simulink model "DY05S600_robot_controller_main_opensource"  (R2020a)
settings: Solver=FixedStepAuto  StartTime=0.0  StopTime=inf  FixedStep=SAMPLE_TIME  RelTol=1e-3
(part 1 of 2)
settings Model: ExplicitPartitioning=on  Creator=86166  LastModifiedBy=win
settings OptimizationCC: BlockReduction=off  EnhancedBackFolding=on  PassReuseOutputArgsThreshold=0  OptimizeBlockOrder=speed  DifferentSizesBufferReuse=on  OptimizationCustomize=off
settings DebuggingCC: ParameterTunabilityLossMsg=error
settings HardwareCC: ProdBitPerLong=64  ProdHWDeviceType=Intel->x86-64 (Linux 64)  TargetBitPerPointer=64  TargetBitPerSizeT=64  TargetBitPerPtrDiffT=64  TargetLongLongMode=on  TargetIntDivRoundTo=Zero  TargetEndianess=LittleEndian  TargetWordSize=64  TargetHWDeviceType=Custom Processor->MATLAB Host Computer
settings RTWCC: Description=Generic Real-Time Target  SystemTargetFile=links_rtlnx_grt.tlc  GenCodeOnly=on  TemplateMakefile=links_rtlnx_grt.tmf  GenerateReport=on  RTWVerbose=off  CustomLibrary=libethercat.a  LaunchReport=on
settings CodeAppCC: ForceParamTrailComments=on  OperatorAnnotations=on
settings STFCustomTargetCC: ModelReferenceCompliant=off  CombineOutputUpdateFcns=on  SystemTargetFile=links_rtlnx_grt.tlc
settings GRTTargetCC: TargetLangStandard=C89/C90 (ANSI)  ModelReferenceCompliant=off  ParMdlRefBuildCompliant=off  CompOptLevelCompliant=off  ConcurrentExecutionCompliant=off  MatFileLogging=off  CPPClassGenCompliant=off  UseToolchainInfoCompliant=off  RTWCAPISignals=on  RTWCAPIParams=on  RTWCAPIRootIO=on

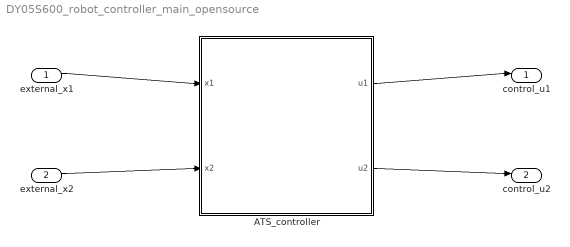
== system DY05S600_robot_controller_main_opensource ==
  external_x1 : Inport
  external_x2 : Inport  Port=2
  ATS_controller : Subsystem
  control_u1 : Outport
  control_u2 : Outport  Port=2
  wires:
  external_x1/1 -> ATS_controller/1(x1)
  external_x2/1 -> ATS_controller/2(x2)
  ATS_controller/1(u1) -> control_u1/1
  ATS_controller/2(u2) -> control_u2/1

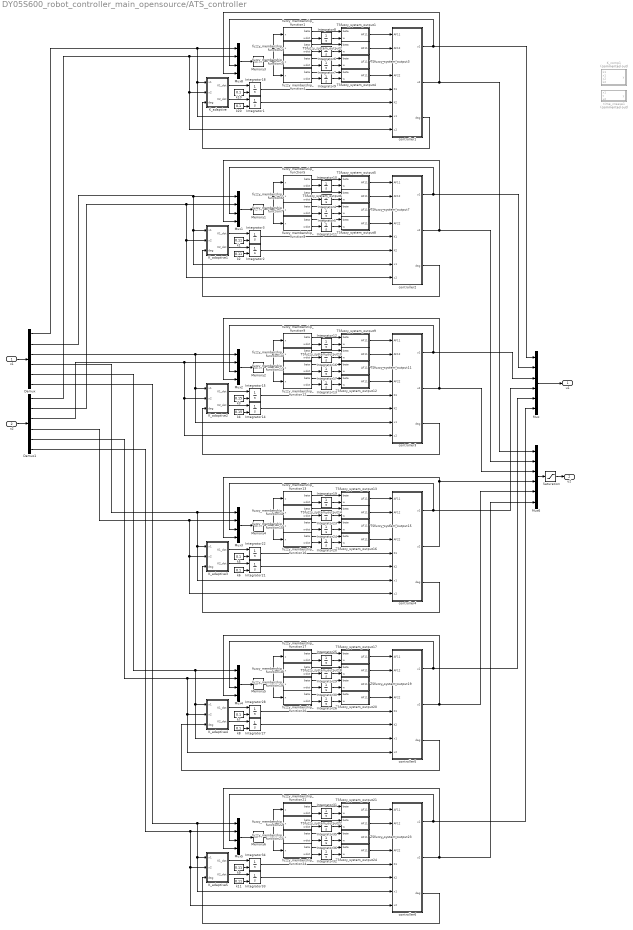
== system DY05S600_robot_controller_main_opensource/ATS_controller ==
  x1 : Inport
  x2 : Inport  Port=2
  Demux : Demux  Outputs=6
  Demux1 : Demux  Outputs=6
  Integrator{1..3,14..15,18,21..22,27..28,33..34} (12 alike) : Integrator  InitialConditionSource=external
  Integrator{4..13,16..17,19..20,23..26,29..32,35..36} (24 alike) : Integrator
  K_adaptive : MATLAB Function  TreatAsAtomicUnit=on
  K_adaptive1 : MATLAB Function  TreatAsAtomicUnit=on
  K_adaptive2 : MATLAB Function  TreatAsAtomicUnit=on
  K_adaptive3 : MATLAB Function  TreatAsAtomicUnit=on
  K_adaptive4 : MATLAB Function  TreatAsAtomicUnit=on
  K_adaptive5 : MATLAB Function  TreatAsAtomicUnit=on
  K_comp1 : MATLAB Function  Commented=on  TreatAsAtomicUnit=on
  Memory{1..6} (6 alike) : Memory
  Mux : Mux  Inputs=6
  Mux{1..5,8} (6 alike) : Mux
  Mux6 : Mux  Inputs=6
  Saturation : Saturate  UpperLimit=80  LowerLimit=-80
  TSfuzzy_system_output1 : MATLAB Function  TreatAsAtomicUnit=on
  TSfuzzy_system_output10 : MATLAB Function  TreatAsAtomicUnit=on
  TSfuzzy_system_output11 : MATLAB Function  TreatAsAtomicUnit=on
  TSfuzzy_system_output12 : MATLAB Function  TreatAsAtomicUnit=on
  TSfuzzy_system_output13 : MATLAB Function  TreatAsAtomicUnit=on
  TSfuzzy_system_output14 : MATLAB Function  TreatAsAtomicUnit=on
  TSfuzzy_system_output15 : MATLAB Function  TreatAsAtomicUnit=on
  TSfuzzy_system_output16 : MATLAB Function  TreatAsAtomicUnit=on
  TSfuzzy_system_output17 : MATLAB Function  TreatAsAtomicUnit=on
  TSfuzzy_system_output18 : MATLAB Function  TreatAsAtomicUnit=on
  TSfuzzy_system_output19 : MATLAB Function  TreatAsAtomicUnit=on
  TSfuzzy_system_output2 : MATLAB Function  TreatAsAtomicUnit=on
  TSfuzzy_system_output20 : MATLAB Function  TreatAsAtomicUnit=on
  TSfuzzy_system_output21 : MATLAB Function  TreatAsAtomicUnit=on
  TSfuzzy_system_output22 : MATLAB Function  TreatAsAtomicUnit=on
  TSfuzzy_system_output23 : MATLAB Function  TreatAsAtomicUnit=on
  TSfuzzy_system_output24 : MATLAB Function  TreatAsAtomicUnit=on
  TSfuzzy_system_output3 : MATLAB Function  TreatAsAtomicUnit=on
  TSfuzzy_system_output4 : MATLAB Function  TreatAsAtomicUnit=on
  TSfuzzy_system_output5 : MATLAB Function  TreatAsAtomicUnit=on
  TSfuzzy_system_output6 : MATLAB Function  TreatAsAtomicUnit=on
  TSfuzzy_system_output7 : MATLAB Function  TreatAsAtomicUnit=on
  TSfuzzy_system_output8 : MATLAB Function  TreatAsAtomicUnit=on
  TSfuzzy_system_output9 : MATLAB Function  TreatAsAtomicUnit=on
  controller1 : MATLAB Function  TreatAsAtomicUnit=on
  controller2 : MATLAB Function  TreatAsAtomicUnit=on
  controller3 : MATLAB Function  TreatAsAtomicUnit=on
  controller4 : MATLAB Function  TreatAsAtomicUnit=on
  controller5 : MATLAB Function  TreatAsAtomicUnit=on
  controller6 : MATLAB Function  TreatAsAtomicUnit=on
  fuzzy_membership_function1 : MATLAB Function  TreatAsAtomicUnit=on
  fuzzy_membership_function10 : MATLAB Function  TreatAsAtomicUnit=on
  fuzzy_membership_function11 : MATLAB Function  TreatAsAtomicUnit=on
  fuzzy_membership_function12 : MATLAB Function  TreatAsAtomicUnit=on
  fuzzy_membership_function13 : MATLAB Function  TreatAsAtomicUnit=on
  fuzzy_membership_function14 : MATLAB Function  TreatAsAtomicUnit=on
  fuzzy_membership_function15 : MATLAB Function  TreatAsAtomicUnit=on
  fuzzy_membership_function16 : MATLAB Function  TreatAsAtomicUnit=on
  fuzzy_membership_function17 : MATLAB Function  TreatAsAtomicUnit=on
  fuzzy_membership_function18 : MATLAB Function  TreatAsAtomicUnit=on
  fuzzy_membership_function19 : MATLAB Function  TreatAsAtomicUnit=on
  fuzzy_membership_function2 : MATLAB Function  TreatAsAtomicUnit=on
  fuzzy_membership_function20 : MATLAB Function  TreatAsAtomicUnit=on
  fuzzy_membership_function21 : MATLAB Function  TreatAsAtomicUnit=on
  fuzzy_membership_function22 : MATLAB Function  TreatAsAtomicUnit=on
  fuzzy_membership_function23 : MATLAB Function  TreatAsAtomicUnit=on
  fuzzy_membership_function24 : MATLAB Function  TreatAsAtomicUnit=on
  fuzzy_membership_function3 : MATLAB Function  TreatAsAtomicUnit=on
  fuzzy_membership_function4 : MATLAB Function  TreatAsAtomicUnit=on
  fuzzy_membership_function5 : MATLAB Function  TreatAsAtomicUnit=on
  fuzzy_membership_function6 : MATLAB Function  TreatAsAtomicUnit=on
  fuzzy_membership_function7 : MATLAB Function  TreatAsAtomicUnit=on
  fuzzy_membership_function8 : MATLAB Function  TreatAsAtomicUnit=on
  fuzzy_membership_function9 : MATLAB Function  TreatAsAtomicUnit=on
  k{1..2,9,11} (4 alike) : Constant  Value=0.11  VectorParams1D=off  SampleTime=-1
  k{5..8,10,20} (6 alike) : Constant  Value=0.1  VectorParams1D=off  SampleTime=-1
  k3 : Constant  Value=0.15  VectorParams1D=off  SampleTime=-1
  k4 : Constant  Value=0.15  VectorParams1D=off  SampleTime=-1
  time_crease1 : MATLAB Function  Commented=on  TreatAsAtomicUnit=on
  u1 : Outport
  u2 : Outport  Port=2
  wires:
  TSfuzzy_system_output1/1(AF11) -> controller1/1(AF11)
  k20/1 -> Integrator1/2
  Memory3/1 -> fuzzy_membership_function4/1(x), fuzzy_membership_function3/1(x), fuzzy_membership_function2/1(x), fuzzy_membership_function1/1(x)
  K_adaptive/2(K2_dot) -> Integrator1/1
  Integrator6/1 -> TSfuzzy_system_output2/2(w)
  Mux8/1 -> Memory3/1
  controller1/1(u1) -> Mux8/3, Mux/1
  TSfuzzy_system_output4/1(AF11) -> controller1/4(AF22)
  Integrator8/1 -> TSfuzzy_system_output1/2(w)
  fuzzy_membership_function1/1(beta) -> TSfuzzy_system_output1/1(beta)
  fuzzy_membership_function2/1(beta) -> TSfuzzy_system_output2/1(beta)
  Integrator9/1 -> TSfuzzy_system_output4/2(w)
  fuzzy_membership_function4/1(beta) -> TSfuzzy_system_output4/1(beta)
  fuzzy_membership_function1/2(wdot) -> Integrator8/1
  fuzzy_membership_function2/2(wdot) -> Integrator6/1
  K_adaptive/1(K1_dot) -> Integrator18/1
  Integrator7/1 -> TSfuzzy_system_output3/2(w)
  TSfuzzy_system_output2/1(AF11) -> controller1/2(AF12)
  fuzzy_membership_function3/2(wdot) -> Integrator7/1
  fuzzy_membership_function4/2(wdot) -> Integrator9/1
  TSfuzzy_system_output3/1(AF11) -> controller1/3(AF21)
  k10/1 -> Integrator18/2
  fuzzy_membership_function3/1(beta) -> TSfuzzy_system_output3/1(beta)
  x1/1 -> Demux/1
  x2/1 -> Demux1/1
  Demux1/1 -> controller1/8(x2), K_adaptive/2(x2), Mux8/2
  controller1/3(dag) -> K_adaptive/3(dag)
  fuzzy_membership_function7/1(beta) -> TSfuzzy_system_output7/1(beta)
  k1/1 -> Integrator3/2
  fuzzy_membership_function8/2(wdot) -> Integrator11/1
  TSfuzzy_system_output7/1(AF11) -> controller2/3(AF21)
  fuzzy_membership_function7/2(wdot) -> Integrator5/1
  fuzzy_membership_function5/2(wdot) -> Integrator10/1
  TSfuzzy_system_output6/1(AF11) -> controller2/2(AF12)
  K_adaptive1/1(K1_dot) -> Integrator3/1
  Integrator5/1 -> TSfuzzy_system_output7/2(w)
  Integrator11/1 -> TSfuzzy_system_output8/2(w)
  fuzzy_membership_function8/1(beta) -> TSfuzzy_system_output8/1(beta)
  fuzzy_membership_function6/1(beta) -> TSfuzzy_system_output6/1(beta)
  controller2/1(u1) -> Mux1/3, Mux/2
  Mux1/1 -> Memory1/1
  fuzzy_membership_function5/1(beta) -> TSfuzzy_system_output5/1(beta)
  controller2/2(u2) -> Mux1/4, Mux6/2
  K_adaptive1/2(K2_dot) -> Integrator2/1
  Integrator10/1 -> TSfuzzy_system_output5/2(w)
  k2/1 -> Integrator2/2
  Integrator4/1 -> TSfuzzy_system_output6/2(w)
  controller2/3(dag) -> K_adaptive1/3(dag)
  Memory1/1 -> fuzzy_membership_function8/1(x), fuzzy_membership_function7/1(x), fuzzy_membership_function6/1(x), fuzzy_membership_function5/1(x)
  fuzzy_membership_function6/2(wdot) -> Integrator4/1
  TSfuzzy_system_output5/1(AF11) -> controller2/1(AF11)
  TSfuzzy_system_output8/1(AF11) -> controller2/4(AF22)
  fuzzy_membership_function9/1(beta) -> TSfuzzy_system_output9/1(beta)
  TSfuzzy_system_output12/1(AF11) -> controller3/4(AF22)
  TSfuzzy_system_output9/1(AF11) -> controller3/1(AF11)
  Memory2/1 -> fuzzy_membership_function12/1(x), fuzzy_membership_function11/1(x), fuzzy_membership_function10/1(x), fuzzy_membership_function9/1(x)
  fuzzy_membership_function10/2(wdot) -> Integrator16/1
  Integrator12/1 -> TSfuzzy_system_output9/2(w)
  Integrator16/1 -> TSfuzzy_system_output10/2(w)
  controller3/2(u2) -> Mux2/4, Mux6/3
  fuzzy_membership_function10/1(beta) -> TSfuzzy_system_output10/1(beta)
  Mux2/1 -> Memory2/1
  fuzzy_membership_function11/2(wdot) -> Integrator17/1
  fuzzy_membership_function9/2(wdot) -> Integrator12/1
  TSfuzzy_system_output11/1(AF11) -> controller3/3(AF21)
  TSfuzzy_system_output10/1(AF11) -> controller3/2(AF12)
  fuzzy_membership_function12/2(wdot) -> Integrator13/1
  fuzzy_membership_function12/1(beta) -> TSfuzzy_system_output12/1(beta)
  Integrator17/1 -> TSfuzzy_system_output11/2(w)
  controller3/1(u1) -> Mux2/3, Mux/3
  K_adaptive2/1(K1_dot) -> Integrator15/1
  fuzzy_membership_function11/1(beta) -> TSfuzzy_system_output11/1(beta)
  Integrator13/1 -> TSfuzzy_system_output12/2(w)
  fuzzy_membership_function13/1(beta) -> TSfuzzy_system_output13/1(beta)
  TSfuzzy_system_output16/1(AF11) -> controller4/4(AF22)
  TSfuzzy_system_output13/1(AF11) -> controller4/1(AF11)
  Memory4/1 -> fuzzy_membership_function16/1(x), fuzzy_membership_function15/1(x), fuzzy_membership_function14/1(x), fuzzy_membership_function13/1(x)
  fuzzy_membership_function14/2(wdot) -> Integrator23/1
  Integrator19/1 -> TSfuzzy_system_output13/2(w)
  controller4/3(dag) -> K_adaptive3/3(dag)
  Integrator23/1 -> TSfuzzy_system_output14/2(w)
  controller4/2(u2) -> Mux6/4, Mux3/4
  fuzzy_membership_function14/1(beta) -> TSfuzzy_system_output14/1(beta)
  Mux3/1 -> Memory4/1
  fuzzy_membership_function15/2(wdot) -> Integrator24/1
  fuzzy_membership_function13/2(wdot) -> Integrator19/1
  TSfuzzy_system_output15/1(AF11) -> controller4/3(AF21)
  TSfuzzy_system_output14/1(AF11) -> controller4/2(AF12)
  fuzzy_membership_function16/2(wdot) -> Integrator20/1
  fuzzy_membership_function16/1(beta) -> TSfuzzy_system_output16/1(beta)
  Integrator24/1 -> TSfuzzy_system_output15/2(w)
  controller4/1(u1) -> Mux/4, Mux3/3
  K_adaptive3/1(K1_dot) -> Integrator22/1
  fuzzy_membership_function15/1(beta) -> TSfuzzy_system_output15/1(beta)
  Integrator20/1 -> TSfuzzy_system_output16/2(w)
  fuzzy_membership_function17/1(beta) -> TSfuzzy_system_output17/1(beta)
  TSfuzzy_system_output20/1(AF11) -> controller5/4(AF22)
  TSfuzzy_system_output17/1(AF11) -> controller5/1(AF11)
  Memory5/1 -> fuzzy_membership_function20/1(x), fuzzy_membership_function19/1(x), fuzzy_membership_function18/1(x), fuzzy_membership_function17/1(x)
  fuzzy_membership_function18/2(wdot) -> Integrator29/1
  Integrator25/1 -> TSfuzzy_system_output17/2(w)
  controller5/3(dag) -> K_adaptive4/3(dag)
  Integrator29/1 -> TSfuzzy_system_output18/2(w)
  controller5/2(u2) -> Mux6/5, Mux4/4
  fuzzy_membership_function18/1(beta) -> TSfuzzy_system_output18/1(beta)
  Mux4/1 -> Memory5/1
  fuzzy_membership_function19/2(wdot) -> Integrator30/1
  fuzzy_membership_function17/2(wdot) -> Integrator25/1
  TSfuzzy_system_output19/1(AF11) -> controller5/3(AF21)
  TSfuzzy_system_output18/1(AF11) -> controller5/2(AF12)
  fuzzy_membership_function20/2(wdot) -> Integrator26/1
  fuzzy_membership_function20/1(beta) -> TSfuzzy_system_output20/1(beta)
  Integrator30/1 -> TSfuzzy_system_output19/2(w)
  controller5/1(u1) -> Mux/5, Mux4/3
  K_adaptive4/1(K1_dot) -> Integrator28/1
  fuzzy_membership_function19/1(beta) -> TSfuzzy_system_output19/1(beta)
  Integrator26/1 -> TSfuzzy_system_output20/2(w)
  fuzzy_membership_function21/1(beta) -> TSfuzzy_system_output21/1(beta)
  TSfuzzy_system_output24/1(AF11) -> controller6/4(AF22)
  TSfuzzy_system_output21/1(AF11) -> controller6/1(AF11)
  Memory6/1 -> fuzzy_membership_function24/1(x), fuzzy_membership_function23/1(x), fuzzy_membership_function22/1(x), fuzzy_membership_function21/1(x)
  fuzzy_membership_function22/2(wdot) -> Integrator35/1
  Integrator31/1 -> TSfuzzy_system_output21/2(w)
  controller6/3(dag) -> K_adaptive5/3(dag)
  Integrator35/1 -> TSfuzzy_system_output22/2(w)
  fuzzy_membership_function22/1(beta) -> TSfuzzy_system_output22/1(beta)
  Mux5/1 -> Memory6/1
  fuzzy_membership_function23/2(wdot) -> Integrator36/1
  fuzzy_membership_function21/2(wdot) -> Integrator31/1
  TSfuzzy_system_output23/1(AF11) -> controller6/3(AF21)
  TSfuzzy_system_output22/1(AF11) -> controller6/2(AF12)
  fuzzy_membership_function24/2(wdot) -> Integrator32/1
  fuzzy_membership_function24/1(beta) -> TSfuzzy_system_output24/1(beta)
  Integrator36/1 -> TSfuzzy_system_output23/2(w)
  controller6/1(u1) -> Mux5/3, Mux/6
  K_adaptive5/1(K1_dot) -> Integrator34/1
  fuzzy_membership_function23/1(beta) -> TSfuzzy_system_output23/1(beta)
  Integrator32/1 -> TSfuzzy_system_output24/2(w)
  Demux/2 -> controller2/7(x1), K_adaptive1/1(x1), Mux1/1
  Demux1/2 -> controller2/8(x2), K_adaptive1/2(x2), Mux1/2
  Demux1/3 -> K_adaptive2/2(x2), controller3/8(x2), Mux2/2
  Demux/4 -> K_adaptive3/1(x1), controller4/7(x1), Mux3/1
  Demux1/4 -> K_adaptive3/2(x2), controller4/8(x2), Mux3/2
  Demux/5 -> K_adaptive4/1(x1), controller5/7(x1), Mux4/1
  Demux1/5 -> K_adaptive4/2(x2), controller5/8(x2), Mux4/2
  Demux/6 -> K_adaptive5/1(x1), controller6/7(x1), Mux5/1
  Demux1/6 -> K_adaptive5/2(x2), controller6/8(x2), Mux5/2
  Mux/1 -> u1/1
  Mux6/1 -> Saturation/1
  Saturation/1 -> u2/1
  Integrator3/1 -> controller2/5(K1)
  Integrator2/1 -> controller2/6(K2)
  Integrator15/1 -> controller3/5(K1)
  k4/1 -> Integrator14/2
  Integrator14/1 -> controller3/6(K2)
  K_adaptive2/2(K2_dot) -> Integrator14/1
  k3/1 -> Integrator15/2
  k6/1 -> Integrator21/2
  k5/1 -> Integrator22/2
  Integrator21/1 -> controller4/6(K2)
  K_adaptive3/2(K2_dot) -> Integrator21/1
  Integrator22/1 -> controller4/5(K1)
  Demux/3 -> controller3/7(x1), K_adaptive2/1(x1), Mux2/1
  controller3/3(dag) -> K_adaptive2/3(dag)
  K_adaptive4/2(K2_dot) -> Integrator27/1
  k7/1 -> Integrator28/2
  k8/1 -> Integrator27/2
  Integrator27/1 -> controller5/6(K2)
  Integrator28/1 -> controller5/5(K1)
  K_adaptive5/2(K2_dot) -> Integrator33/1
  k9/1 -> Integrator34/2
  k11/1 -> Integrator33/2
  controller6/2(u2) -> Mux6/6, Mux5/4
  controller1/2(u2) -> Mux6/1, Mux8/4
  Demux/1 -> controller1/7(x1), K_adaptive/1(x1), Mux8/1
  Integrator18/1 -> controller1/5(K1)
  Integrator1/1 -> controller1/6(K2)
  Integrator34/1 -> controller6/5(K1)
  Integrator33/1 -> controller6/6(K2)

== matlab function DY05S600_robot_controller_main_opensource/ATS_controller/fuzzy_membership_function22 ==
  data: x input; beta output; wdot output
function [beta,wdot] = fcn(x)

%xm是规则中心
xm=zeros(5,4);
for j=1:5
    xm(j,1)=-0.26+0.13*(j-1)+0.1;
end
for j=6:10
    xm(j-5,2)=-0.18+0.09*(j-5-1)+0.1;
end
for j=11:15
    xm(j-10,3)=-0.14+0.07*(j-10-1)+0.1;
end
for j=16:20
    xm(j-15,4)=-0.4+0.2*(j-15-1)+0.1;
end



%xm是规则中心从小值到大值排列,x是前件变量,
r=length(xm(:,1)); %length(xm)是规则数量r
n=length(xm(1,:));%length(x)是前件变量维度
%初始化隶属度函数
ux=zeros(r,n);

for k=1:n
    if x(k)<=xm(1,k)   %论域左边界外
        ux(1,k)=1;
    end
    if x(k)>=xm(r,k)   %论域右边界外
        ux(r,k)=1;
    end
    for i=1:r-1  %从左到右只计算下降的隶属度函数
        if x(k)>=xm(i,k)&&x(k)<=xm(i+1,k)
           ux(i,k)=0.5*sin(pi*(x(k)-xm(i,k))/abs(xm(i,k)-xm(i+1,k))+0.5*pi)+0.5; %一种具有一阶可导性的四边形家族隶属度函数
        end
    end
    for i=2:r  %从左到右只计算上升的隶属度函数
        if x(k)>=xm(i-1,k)&&x(k)<=xm(i,k)
           ux(i,k)=0.5*sin(pi*(x(k)-xm(i,k))/abs(xm(i-1,k)-xm(i,k))+0.5*pi)+0.5;
        end
    end
end

kx=1;
jz=1;
[beta,wdot]= fuzzyoutput(ux,x,xm,kx,jz);

% function  [Basic,beta]= sumfuzzy_test(x) 
% ux=x;
% im=1;
% jm=0;
% bias=1;
% Basic=0;
% dem=length(ux(:,1))^length(ux(1,:)); %隶属度函数的重数数量
% beta=zeros(dem,1);
% [Basic,beta] = myfun(im,jm,ux,bias,Basic,beta);
% function [Basic,beta,jm] = myfun(im,jm,ux,bias,Basic,beta) 
% %针对ux隶属度函数矩阵的中心平均解模糊，初值赋为1,0，ux，1，0，执行的是多重求和
%     if  im > length(ux(1,:))    %length(ux(1,:))为前件输入的维度
%         Basic = Basic + bias;
%         jm=jm+1;                %相对于i1...in规则编号，此处是从最后一列填满到第一列（i1,...,in）
%         beta(jm,1)=bias;        %beta(i1,...,in)*xk*z(i6,j)
%     else
%         for km=1:length(ux(:,1))   %length(ux(:,1))为规则数量
%             bias_last = bias;
%             bias = bias* ux(km,im);
%             im = im+1;
%             [Basic,beta,jm] = myfun(im,jm,ux,bias,Basic,beta); %递归，拦在这里一直到function执行结束,每执行一次就会多一个for循环（每次跳出就是再一次的for内循环）
%             im = im-1; 
%             bias  = bias_last;
%         end
%     end
% end


end

== matlab function DY05S600_robot_controller_main_opensource/ATS_controller/fuzzy_membership_function23 ==
  data: x input; beta output; wdot output
function [beta,wdot] = fcn(x)

%xm是规则中心
xm=zeros(5,4);
for j=1:5
    xm(j,1)=-0.26+0.13*(j-1)+0.1;
end
for j=6:10
    xm(j-5,2)=-0.18+0.09*(j-5-1)+0.1;
end
for j=11:15
    xm(j-10,3)=-0.14+0.07*(j-10-1)+0.1;
end
for j=16:20
    xm(j-15,4)=-0.4+0.2*(j-15-1)+0.1;
end


%xm是规则中心从小值到大值排列,x是前件变量,
r=length(xm(:,1)); %length(xm)是规则数量r
n=length(xm(1,:));%length(x)是前件变量维度
%初始化隶属度函数
ux=zeros(r,n);

for k=1:n
    if x(k)<=xm(1,k)   %论域左边界外
        ux(1,k)=1;
    end
    if x(k)>=xm(r,k)   %论域右边界外
        ux(r,k)=1;
    end
    for i=1:r-1  %从左到右只计算下降的隶属度函数
        if x(k)>=xm(i,k)&&x(k)<=xm(i+1,k)
           ux(i,k)=0.5*sin(pi*(x(k)-xm(i,k))/abs(xm(i,k)-xm(i+1,k))+0.5*pi)+0.5; %一种具有一阶可导性的四边形家族隶属度函数
        end
    end
    for i=2:r  %从左到右只计算上升的隶属度函数
        if x(k)>=xm(i-1,k)&&x(k)<=xm(i,k)
           ux(i,k)=0.5*sin(pi*(x(k)-xm(i,k))/abs(xm(i-1,k)-xm(i,k))+0.5*pi)+0.5;
        end
    end
end

kx=1;
jz=1;
[beta,wdot]= fuzzyoutput(ux,x,xm,kx,jz);

% function  [Basic,beta]= sumfuzzy_test(x) 
% ux=x;
% im=1;
% jm=0;
% bias=1;
% Basic=0;
% dem=length(ux(:,1))^length(ux(1,:)); %隶属度函数的重数数量
% beta=zeros(dem,1);
% [Basic,beta] = myfun(im,jm,ux,bias,Basic,beta);
% function [Basic,beta,jm] = myfun(im,jm,ux,bias,Basic,beta) 
% %针对ux隶属度函数矩阵的中心平均解模糊，初值赋为1,0，ux，1，0，执行的是多重求和
%     if  im > length(ux(1,:))    %length(ux(1,:))为前件输入的维度
%         Basic = Basic + bias;
%         jm=jm+1;                %相对于i1...in规则编号，此处是从最后一列填满到第一列（i1,...,in）
%         beta(jm,1)=bias;        %beta(i1,...,in)*xk*z(i6,j)
%     else
%         for km=1:length(ux(:,1))   %length(ux(:,1))为规则数量
%             bias_last = bias;
%             bias = bias* ux(km,im);
%             im = im+1;
%             [Basic,beta,jm] = myfun(im,jm,ux,bias,Basic,beta); %递归，拦在这里一直到function执行结束,每执行一次就会多一个for循环（每次跳出就是再一次的for内循环）
%             im = im-1; 
%             bias  = bias_last;
%         end
%     end
% end


end

== matlab function DY05S600_robot_controller_main_opensource/ATS_controller/fuzzy_membership_function24 ==
  data: x input; beta output; wdot output
function [beta,wdot] = fcn(x)

%xm是规则中心
xm=zeros(5,4);
for j=1:5
    xm(j,1)=-0.26+0.13*(j-1)+0.1;
end
for j=6:10
    xm(j-5,2)=-0.18+0.09*(j-5-1)+0.1;
end
for j=11:15
    xm(j-10,3)=-0.14+0.07*(j-10-1)+0.1;
end
for j=16:20
    xm(j-15,4)=-0.4+0.2*(j-15-1)+0.1;
end



%xm是规则中心从小值到大值排列,x是前件变量,
r=length(xm(:,1)); %length(xm)是规则数量r
n=length(xm(1,:));%length(x)是前件变量维度
%初始化隶属度函数
ux=zeros(r,n);

for k=1:n
    if x(k)<=xm(1,k)   %论域左边界外
        ux(1,k)=1;
    end
    if x(k)>=xm(r,k)   %论域右边界外
        ux(r,k)=1;
    end
    for i=1:r-1  %从左到右只计算下降的隶属度函数
        if x(k)>=xm(i,k)&&x(k)<=xm(i+1,k)
           ux(i,k)=0.5*sin(pi*(x(k)-xm(i,k))/abs(xm(i,k)-xm(i+1,k))+0.5*pi)+0.5; %一种具有一阶可导性的四边形家族隶属度函数
        end
    end
    for i=2:r  %从左到右只计算上升的隶属度函数
        if x(k)>=xm(i-1,k)&&x(k)<=xm(i,k)
           ux(i,k)=0.5*sin(pi*(x(k)-xm(i,k))/abs(xm(i-1,k)-xm(i,k))+0.5*pi)+0.5;
        end
    end
end

kx=1;
jz=1;
[beta,wdot]= fuzzyoutput(ux,x,xm,kx,jz);

% function  [Basic,beta]= sumfuzzy_test(x) 
% ux=x;
% im=1;
% jm=0;
% bias=1;
% Basic=0;
% dem=length(ux(:,1))^length(ux(1,:)); %隶属度函数的重数数量
% beta=zeros(dem,1);
% [Basic,beta] = myfun(im,jm,ux,bias,Basic,beta);
% function [Basic,beta,jm] = myfun(im,jm,ux,bias,Basic,beta) 
% %针对ux隶属度函数矩阵的中心平均解模糊，初值赋为1,0，ux，1，0，执行的是多重求和
%     if  im > length(ux(1,:))    %length(ux(1,:))为前件输入的维度
%         Basic = Basic + bias;
%         jm=jm+1;                %相对于i1...in规则编号，此处是从最后一列填满到第一列（i1,...,in）
%         beta(jm,1)=bias;        %beta(i1,...,in)*xk*z(i6,j)
%     else
%         for km=1:length(ux(:,1))   %length(ux(:,1))为规则数量
%             bias_last = bias;
%             bias = bias* ux(km,im);
%             im = im+1;
%             [Basic,beta,jm] = myfun(im,jm,ux,bias,Basic,beta); %递归，拦在这里一直到function执行结束,每执行一次就会多一个for循环（每次跳出就是再一次的for内循环）
%             im = im-1; 
%             bias  = bias_last;
%         end
%     end
% end


end

== matlab function DY05S600_robot_controller_main_opensource/ATS_controller/K_adaptive3 ==
  data: K1_dot output; x1 input; x2 input; dag input; K2_dot output
function [K1_dot,K2_dot]  = fcn(x1,x2,dag)
w1=0.0001;
w2=0.0001;
K1_dot=w1*x1*4/pi*atan(x1/dag);
K2_dot=w2*x2*4/pi*atan(x2/dag);
end

== matlab function DY05S600_robot_controller_main_opensource/ATS_controller/time_crease1 ==
  data: y output; x1 input; t input; x2 input
function y   = fcn(x1,t,x2)
y1=2/pi*(atan(2*t-1)+pi/4)*x1;
y2=2/pi*(atan(2*t-1)+pi/4)*x2;
y=[y1,y2]';
end

== matlab function DY05S600_robot_controller_main_opensource/ATS_controller/K_adaptive4 ==
  data: K1_dot output; x1 input; x2 input; dag input; K2_dot output
function [K1_dot,K2_dot]  = fcn(x1,x2,dag)
w1=0.0001;
w2=0.0001;
K1_dot=w1*x1*4/pi*atan(x1/dag);
K2_dot=w2*x2*4/pi*atan(x2/dag);
end

== matlab function DY05S600_robot_controller_main_opensource/ATS_controller/K_adaptive5 ==
  data: K1_dot output; x1 input; x2 input; dag input; K2_dot output
function [K1_dot,K2_dot]  = fcn(x1,x2,dag)

w1=0.0001;
w2=0.0001;

K1_dot=w1*x1*4/pi*atan(x1/dag);
K2_dot=w2*x2*4/pi*atan(x2/dag);

end

== matlab function DY05S600_robot_controller_main_opensource/ATS_controller/K_adaptive2 ==
  data: K1_dot output; x1 input; x2 input; dag input; K2_dot output
function [K1_dot,K2_dot]  = fcn(x1,x2,dag)
w1=0.0001;
w2=0.0001;
K1_dot=w1*x1*4/pi*atan(x1/dag);
K2_dot=w2*x2*4/pi*atan(x2/dag);
end

== matlab function DY05S600_robot_controller_main_opensource/ATS_controller/K_adaptive1 ==
  data: K1_dot output; x1 input; x2 input; dag input; K2_dot output
function [K1_dot,K2_dot]  = fcn(x1,x2,dag)
w1=0.0001;
w2=0.0001;
K1_dot=w1*x1*4/pi*atan(x1/dag);
K2_dot=w2*x2*4/pi*atan(x2/dag);
end

== matlab function DY05S600_robot_controller_main_opensource/ATS_controller/TSfuzzy_system_output5 ==
  data: beta input; w input; AF11 output
function AF11  = fcn(beta,w)

AF11=0;
for i=1:length(beta)
    AF11=AF11+w(i,1)*beta(i,1);
end

end

== matlab function DY05S600_robot_controller_main_opensource/ATS_controller/TSfuzzy_system_output6 ==
  data: beta input; w input; AF11 output
function AF11  = fcn(beta,w)

AF11=0;
for i=1:length(beta)
    AF11=AF11+w(i,1)*beta(i,1);
end

end

== matlab function DY05S600_robot_controller_main_opensource/ATS_controller/K_adaptive ==
  data: K1_dot output; x1 input; x2 input; dag input; K2_dot output
function [K1_dot,K2_dot]  = fcn(x1,x2,dag)
w1=0.0001;
w2=0.0001;
K1_dot=w1*x1*4/pi*atan(x1/dag);
K2_dot=w2*x2*4/pi*atan(x2/dag);
end

== matlab function DY05S600_robot_controller_main_opensource/ATS_controller/TSfuzzy_system_output1 ==
  data: beta input; w input; AF11 output
function AF11  = fcn(beta,w)

AF11=0;
for i=1:length(beta)
    AF11=AF11+w(i,1)*beta(i,1);
end

end

== matlab function DY05S600_robot_controller_main_opensource/ATS_controller/TSfuzzy_system_output2 ==
  data: beta input; w input; AF11 output
function AF11  = fcn(beta,w)

AF11=0;
for i=1:length(beta)
    AF11=AF11+w(i,1)*beta(i,1);
end

end

== matlab function DY05S600_robot_controller_main_opensource/ATS_controller/TSfuzzy_system_output3 ==
  data: beta input; w input; AF11 output
function AF11  = fcn(beta,w)

AF11=0;
for i=1:length(beta)
    AF11=AF11+w(i,1)*beta(i,1);
end

end

== matlab function DY05S600_robot_controller_main_opensource/ATS_controller/TSfuzzy_system_output4 ==
  data: beta input; w input; AF11 output
function AF11  = fcn(beta,w)

AF11=0;
for i=1:length(beta)
    AF11=AF11+w(i,1)*beta(i,1);
end

end

== matlab function DY05S600_robot_controller_main_opensource/ATS_controller/controller1 ==
  data: AF11 input; AF12 input; AF21 input; AF22 input; K1 input; K2 input; u1 output; u2 output; x1 input; x2 input; dag output
function [u1,u2,dag]  = fcn(AF11,AF12,AF21,AF22,K1,K2,x1,x2)

b1=0.1;
b2=0.01;

dag=1*pi/180;

% u1=-1/b1*((0+AF11)*x1+(0+AF12)*x2+K1*x1/dag^2);
% 
% u2=-1/b2*((0+AF21)*x1+(0+AF22)*x2+K2*x2/dag^2);

% dagx1=0.5*pi/180;
% satx1=0;
% if abs(x1)<dagx1
%     satx1=sign(x1);
% else
%     satx1=x1/dagx1;
% end

   
u1=-1/b1*((0.2+AF11)*x1+(0+AF12)*x2+K1*4/pi*atan(x1/dag));

u2=-1/b2*((2+AF21)*x1+(0.2+AF22)*x2+K2*4/pi*atan(x2/dag));


end

== matlab function DY05S600_robot_controller_main_opensource/ATS_controller/TSfuzzy_system_output7 ==
  data: beta input; w input; AF11 output
function AF11  = fcn(beta,w)

AF11=0;
for i=1:length(beta)
    AF11=AF11+w(i,1)*beta(i,1);
end

end

== matlab function DY05S600_robot_controller_main_opensource/ATS_controller/fuzzy_membership_function1 ==
  data: x input; beta output; wdot output
function [beta,wdot] = fcn(x)

%xm是规则中心
xm=zeros(5,4);
for j=1:5
    xm(j,1)=-0.26+0.13*(j-1)+0.1;
end
for j=6:10
    xm(j-5,2)=-0.18+0.09*(j-5-1)+0.1;
end
for j=11:15
    xm(j-10,3)=-0.14+0.07*(j-10-1)+0.1;
end
for j=16:20
    xm(j-15,4)=-0.4+0.2*(j-15-1)+0.1;
end



%xm是规则中心从小值到大值排列,x是前件变量,
r=length(xm(:,1)); %length(xm)是规则数量r
n=length(xm(1,:));%length(x)是前件变量维度
%初始化隶属度函数
ux=zeros(r,n);

for k=1:n
    if x(k)<=xm(1,k)   %论域左边界外
        ux(1,k)=1;
    end
    if x(k)>=xm(r,k)   %论域右边界外
        ux(r,k)=1;
    end
    for i=1:r-1  %从左到右只计算下降的隶属度函数
        if x(k)>=xm(i,k)&&x(k)<=xm(i+1,k)
           ux(i,k)=0.5*sin(pi*(x(k)-xm(i,k))/abs(xm(i,k)-xm(i+1,k))+0.5*pi)+0.5; %一种具有一阶可导性的四边形家族隶属度函数
        end
    end
    for i=2:r  %从左到右只计算上升的隶属度函数
        if x(k)>=xm(i-1,k)&&x(k)<=xm(i,k)
           ux(i,k)=0.5*sin(pi*(x(k)-xm(i,k))/abs(xm(i-1,k)-xm(i,k))+0.5*pi)+0.5;
        end
    end
end

kx=1;
jz=1;
[beta,wdot]= fuzzyoutput(ux,x,xm,kx,jz);

% function  [Basic,beta]= sumfuzzy_test(x) 
% ux=x;
% im=1;
% jm=0;
% bias=1;
% Basic=0;
% dem=length(ux(:,1))^length(ux(1,:)); %隶属度函数的重数数量
% beta=zeros(dem,1);
% [Basic,beta] = myfun(im,jm,ux,bias,Basic,beta);
% function [Basic,beta,jm] = myfun(im,jm,ux,bias,Basic,beta) 
% %针对ux隶属度函数矩阵的中心平均解模糊，初值赋为1,0，ux，1，0，执行的是多重求和
%     if  im > length(ux(1,:))    %length(ux(1,:))为前件输入的维度
%         Basic = Basic + bias;
%         jm=jm+1;                %相对于i1...in规则编号，此处是从最后一列填满到第一列（i1,...,in）
%         beta(jm,1)=bias;        %beta(i1,...,in)*xk*z(i6,j)
%     else
%         for km=1:length(ux(:,1))   %length(ux(:,1))为规则数量
%             bias_last = bias;
%             bias = bias* ux(km,im);
%             im = im+1;
%             [Basic,beta,jm] = myfun(im,jm,ux,bias,Basic,beta); %递归，拦在这里一直到function执行结束,每执行一次就会多一个for循环（每次跳出就是再一次的for内循环）
%             im = im-1; 
%             bias  = bias_last;
%         end
%     end
% end


end

== matlab function DY05S600_robot_controller_main_opensource/ATS_controller/fuzzy_membership_function2 ==
  data: x input; beta output; wdot output
function [beta,wdot] = fcn(x)

%xm是规则中心
xm=zeros(5,4);
for j=1:5
    xm(j,1)=-0.26+0.13*(j-1)+0.1;
end
for j=6:10
    xm(j-5,2)=-0.18+0.09*(j-5-1)+0.1;
end
for j=11:15
    xm(j-10,3)=-0.14+0.07*(j-10-1)+0.1;
end
for j=16:20
    xm(j-15,4)=-0.4+0.2*(j-15-1)+0.1;
end



%xm是规则中心从小值到大值排列,x是前件变量,
r=length(xm(:,1)); %length(xm)是规则数量r
n=length(xm(1,:));%length(x)是前件变量维度
%初始化隶属度函数
ux=zeros(r,n);

for k=1:n
    if x(k)<=xm(1,k)   %论域左边界外
        ux(1,k)=1;
    end
    if x(k)>=xm(r,k)   %论域右边界外
        ux(r,k)=1;
    end
    for i=1:r-1  %从左到右只计算下降的隶属度函数
        if x(k)>=xm(i,k)&&x(k)<=xm(i+1,k)
           ux(i,k)=0.5*sin(pi*(x(k)-xm(i,k))/abs(xm(i,k)-xm(i+1,k))+0.5*pi)+0.5; %一种具有一阶可导性的四边形家族隶属度函数
        end
    end
    for i=2:r  %从左到右只计算上升的隶属度函数
        if x(k)>=xm(i-1,k)&&x(k)<=xm(i,k)
           ux(i,k)=0.5*sin(pi*(x(k)-xm(i,k))/abs(xm(i-1,k)-xm(i,k))+0.5*pi)+0.5;
        end
    end
end

kx=1;
jz=1;
[beta,wdot]= fuzzyoutput(ux,x,xm,kx,jz);

% function  [Basic,beta]= sumfuzzy_test(x) 
% ux=x;
% im=1;
% jm=0;
% bias=1;
% Basic=0;
% dem=length(ux(:,1))^length(ux(1,:)); %隶属度函数的重数数量
% beta=zeros(dem,1);
% [Basic,beta] = myfun(im,jm,ux,bias,Basic,beta);
% function [Basic,beta,jm] = myfun(im,jm,ux,bias,Basic,beta) 
% %针对ux隶属度函数矩阵的中心平均解模糊，初值赋为1,0，ux，1，0，执行的是多重求和
%     if  im > length(ux(1,:))    %length(ux(1,:))为前件输入的维度
%         Basic = Basic + bias;
%         jm=jm+1;                %相对于i1...in规则编号，此处是从最后一列填满到第一列（i1,...,in）
%         beta(jm,1)=bias;        %beta(i1,...,in)*xk*z(i6,j)
%     else
%         for km=1:length(ux(:,1))   %length(ux(:,1))为规则数量
%             bias_last = bias;
%             bias = bias* ux(km,im);
%             im = im+1;
%             [Basic,beta,jm] = myfun(im,jm,ux,bias,Basic,beta); %递归，拦在这里一直到function执行结束,每执行一次就会多一个for循环（每次跳出就是再一次的for内循环）
%             im = im-1; 
%             bias  = bias_last;
%         end
%     end
% end


end

== matlab function DY05S600_robot_controller_main_opensource/ATS_controller/fuzzy_membership_function3 ==
  data: x input; beta output; wdot output
function [beta,wdot] = fcn(x)

%xm是规则中心
xm=zeros(5,4);
for j=1:5
    xm(j,1)=-0.26+0.13*(j-1)+0.1;
end
for j=6:10
    xm(j-5,2)=-0.18+0.09*(j-5-1)+0.1;
end
for j=11:15
    xm(j-10,3)=-0.14+0.07*(j-10-1)+0.1;
end
for j=16:20
    xm(j-15,4)=-0.4+0.2*(j-15-1)+0.1;
end


%xm是规则中心从小值到大值排列,x是前件变量,
r=length(xm(:,1)); %length(xm)是规则数量r
n=length(xm(1,:));%length(x)是前件变量维度
%初始化隶属度函数
ux=zeros(r,n);

for k=1:n
    if x(k)<=xm(1,k)   %论域左边界外
        ux(1,k)=1;
    end
    if x(k)>=xm(r,k)   %论域右边界外
        ux(r,k)=1;
    end
    for i=1:r-1  %从左到右只计算下降的隶属度函数
        if x(k)>=xm(i,k)&&x(k)<=xm(i+1,k)
           ux(i,k)=0.5*sin(pi*(x(k)-xm(i,k))/abs(xm(i,k)-xm(i+1,k))+0.5*pi)+0.5; %一种具有一阶可导性的四边形家族隶属度函数
        end
    end
    for i=2:r  %从左到右只计算上升的隶属度函数
        if x(k)>=xm(i-1,k)&&x(k)<=xm(i,k)
           ux(i,k)=0.5*sin(pi*(x(k)-xm(i,k))/abs(xm(i-1,k)-xm(i,k))+0.5*pi)+0.5;
        end
    end
end

kx=1;
jz=1;
[beta,wdot]= fuzzyoutput(ux,x,xm,kx,jz);

% function  [Basic,beta]= sumfuzzy_test(x) 
% ux=x;
% im=1;
% jm=0;
% bias=1;
% Basic=0;
% dem=length(ux(:,1))^length(ux(1,:)); %隶属度函数的重数数量
% beta=zeros(dem,1);
% [Basic,beta] = myfun(im,jm,ux,bias,Basic,beta);
% function [Basic,beta,jm] = myfun(im,jm,ux,bias,Basic,beta) 
% %针对ux隶属度函数矩阵的中心平均解模糊，初值赋为1,0，ux，1，0，执行的是多重求和
%     if  im > length(ux(1,:))    %length(ux(1,:))为前件输入的维度
%         Basic = Basic + bias;
%         jm=jm+1;                %相对于i1...in规则编号，此处是从最后一列填满到第一列（i1,...,in）
%         beta(jm,1)=bias;        %beta(i1,...,in)*xk*z(i6,j)
%     else
%         for km=1:length(ux(:,1))   %length(ux(:,1))为规则数量
%             bias_last = bias;
%             bias = bias* ux(km,im);
%             im = im+1;
%             [Basic,beta,jm] = myfun(im,jm,ux,bias,Basic,beta); %递归，拦在这里一直到function执行结束,每执行一次就会多一个for循环（每次跳出就是再一次的for内循环）
%             im = im-1; 
%             bias  = bias_last;
%         end
%     end
% end


end

== matlab function DY05S600_robot_controller_main_opensource/ATS_controller/fuzzy_membership_function4 ==
  data: x input; beta output; wdot output
function [beta,wdot] = fcn(x)

%xm是规则中心
xm=zeros(5,4);
for j=1:5
    xm(j,1)=-0.26+0.13*(j-1)+0.1;
end
for j=6:10
    xm(j-5,2)=-0.18+0.09*(j-5-1)+0.1;
end
for j=11:15
    xm(j-10,3)=-0.14+0.07*(j-10-1)+0.1;
end
for j=16:20
    xm(j-15,4)=-0.4+0.2*(j-15-1)+0.1;
end



%xm是规则中心从小值到大值排列,x是前件变量,
r=length(xm(:,1)); %length(xm)是规则数量r
n=length(xm(1,:));%length(x)是前件变量维度
%初始化隶属度函数
ux=zeros(r,n);

for k=1:n
    if x(k)<=xm(1,k)   %论域左边界外
        ux(1,k)=1;
    end
    if x(k)>=xm(r,k)   %论域右边界外
        ux(r,k)=1;
    end
    for i=1:r-1  %从左到右只计算下降的隶属度函数
        if x(k)>=xm(i,k)&&x(k)<=xm(i+1,k)
           ux(i,k)=0.5*sin(pi*(x(k)-xm(i,k))/abs(xm(i,k)-xm(i+1,k))+0.5*pi)+0.5; %一种具有一阶可导性的四边形家族隶属度函数
        end
    end
    for i=2:r  %从左到右只计算上升的隶属度函数
        if x(k)>=xm(i-1,k)&&x(k)<=xm(i,k)
           ux(i,k)=0.5*sin(pi*(x(k)-xm(i,k))/abs(xm(i-1,k)-xm(i,k))+0.5*pi)+0.5;
        end
    end
end

kx=1;
jz=1;
[beta,wdot]= fuzzyoutput(ux,x,xm,kx,jz);

% function  [Basic,beta]= sumfuzzy_test(x) 
% ux=x;
% im=1;
% jm=0;
% bias=1;
% Basic=0;
% dem=length(ux(:,1))^length(ux(1,:)); %隶属度函数的重数数量
% beta=zeros(dem,1);
% [Basic,beta] = myfun(im,jm,ux,bias,Basic,beta);
% function [Basic,beta,jm] = myfun(im,jm,ux,bias,Basic,beta) 
% %针对ux隶属度函数矩阵的中心平均解模糊，初值赋为1,0，ux，1，0，执行的是多重求和
%     if  im > length(ux(1,:))    %length(ux(1,:))为前件输入的维度
%         Basic = Basic + bias;
%         jm=jm+1;                %相对于i1...in规则编号，此处是从最后一列填满到第一列（i1,...,in）
%         beta(jm,1)=bias;        %beta(i1,...,in)*xk*z(i6,j)
%     else
%         for km=1:length(ux(:,1))   %length(ux(:,1))为规则数量
%             bias_last = bias;
%             bias = bias* ux(km,im);
%             im = im+1;
%             [Basic,beta,jm] = myfun(im,jm,ux,bias,Basic,beta); %递归，拦在这里一直到function执行结束,每执行一次就会多一个for循环（每次跳出就是再一次的for内循环）
%             im = im-1; 
%             bias  = bias_last;
%         end
%     end
% end


end

== matlab function DY05S600_robot_controller_main_opensource/ATS_controller/TSfuzzy_system_output8 ==
  data: beta input; w input; AF11 output
function AF11  = fcn(beta,w)

AF11=0;
for i=1:length(beta)
    AF11=AF11+w(i,1)*beta(i,1);
end

end

== matlab function DY05S600_robot_controller_main_opensource/ATS_controller/controller2 ==
  data: AF11 input; AF12 input; AF21 input; AF22 input; K1 input; K2 input; u1 output; u2 output; x1 input; x2 input; dag output
function [u1,u2,dag]  = fcn(AF11,AF12,AF21,AF22,K1,K2,x1,x2)

b1=0.1;
b2=0.01;

dag=1.2*pi/180;

% u1=-1/b1*((0+AF11)*x1+(0+AF12)*x2+K1*x1/dag^2);
% 
% u2=-1/b2*((0+AF21)*x1+(0+AF22)*x2+K2*x2/dag^2);

% dagx1=0.5*pi/180;
% satx1=0;
% if abs(x1)<dagx1
%     satx1=sign(x1);
% else
%     satx1=x1/dagx1;
% end

   
u1=-1/b1*((0.5+AF11)*x1+(0+AF12)*x2+K1*4/pi*atan(x1/dag));

u2=-1/b2*((2+AF21)*x1+(0.5+AF22)*x2+K2*4/pi*atan(x2/dag));

end

== matlab function DY05S600_robot_controller_main_opensource/ATS_controller/fuzzy_membership_function5 ==
  data: x input; beta output; wdot output
function [beta,wdot] = fcn(x)

%xm是规则中心
xm=zeros(5,4);
for j=1:5
    xm(j,1)=-0.26+0.13*(j-1)+0.1;
end
for j=6:10
    xm(j-5,2)=-0.18+0.09*(j-5-1)+0.1;
end
for j=11:15
    xm(j-10,3)=-0.14+0.07*(j-10-1)+0.1;
end
for j=16:20
    xm(j-15,4)=-0.4+0.2*(j-15-1)+0.1;
end



%xm是规则中心从小值到大值排列,x是前件变量,
r=length(xm(:,1)); %length(xm)是规则数量r
n=length(xm(1,:));%length(x)是前件变量维度
%初始化隶属度函数
ux=zeros(r,n);

for k=1:n
    if x(k)<=xm(1,k)   %论域左边界外
        ux(1,k)=1;
    end
    if x(k)>=xm(r,k)   %论域右边界外
        ux(r,k)=1;
    end
    for i=1:r-1  %从左到右只计算下降的隶属度函数
        if x(k)>=xm(i,k)&&x(k)<=xm(i+1,k)
           ux(i,k)=0.5*sin(pi*(x(k)-xm(i,k))/abs(xm(i,k)-xm(i+1,k))+0.5*pi)+0.5; %一种具有一阶可导性的四边形家族隶属度函数
        end
    end
    for i=2:r  %从左到右只计算上升的隶属度函数
        if x(k)>=xm(i-1,k)&&x(k)<=xm(i,k)
           ux(i,k)=0.5*sin(pi*(x(k)-xm(i,k))/abs(xm(i-1,k)-xm(i,k))+0.5*pi)+0.5;
        end
    end
end

kx=1;
jz=1;
[beta,wdot]= fuzzyoutput(ux,x,xm,kx,jz);

% function  [Basic,beta]= sumfuzzy_test(x) 
% ux=x;
% im=1;
% jm=0;
% bias=1;
% Basic=0;
% dem=length(ux(:,1))^length(ux(1,:)); %隶属度函数的重数数量
% beta=zeros(dem,1);
% [Basic,beta] = myfun(im,jm,ux,bias,Basic,beta);
% function [Basic,beta,jm] = myfun(im,jm,ux,bias,Basic,beta) 
% %针对ux隶属度函数矩阵的中心平均解模糊，初值赋为1,0，ux，1，0，执行的是多重求和
%     if  im > length(ux(1,:))    %length(ux(1,:))为前件输入的维度
%         Basic = Basic + bias;
%         jm=jm+1;                %相对于i1...in规则编号，此处是从最后一列填满到第一列（i1,...,in）
%         beta(jm,1)=bias;        %beta(i1,...,in)*xk*z(i6,j)
%     else
%         for km=1:length(ux(:,1))   %length(ux(:,1))为规则数量
%             bias_last = bias;
%             bias = bias* ux(km,im);
%             im = im+1;
%             [Basic,beta,jm] = myfun(im,jm,ux,bias,Basic,beta); %递归，拦在这里一直到function执行结束,每执行一次就会多一个for循环（每次跳出就是再一次的for内循环）
%             im = im-1; 
%             bias  = bias_last;
%         end
%     end
% end


end

== matlab function DY05S600_robot_controller_main_opensource/ATS_controller/fuzzy_membership_function6 ==
  data: x input; beta output; wdot output
function [beta,wdot] = fcn(x)

%xm是规则中心
xm=zeros(5,4);
for j=1:5
    xm(j,1)=-0.26+0.13*(j-1)+0.1;
end
for j=6:10
    xm(j-5,2)=-0.18+0.09*(j-5-1)+0.1;
end
for j=11:15
    xm(j-10,3)=-0.14+0.07*(j-10-1)+0.1;
end
for j=16:20
    xm(j-15,4)=-0.4+0.2*(j-15-1)+0.1;
end



%xm是规则中心从小值到大值排列,x是前件变量,
r=length(xm(:,1)); %length(xm)是规则数量r
n=length(xm(1,:));%length(x)是前件变量维度
%初始化隶属度函数
ux=zeros(r,n);

for k=1:n
    if x(k)<=xm(1,k)   %论域左边界外
        ux(1,k)=1;
    end
    if x(k)>=xm(r,k)   %论域右边界外
        ux(r,k)=1;
    end
    for i=1:r-1  %从左到右只计算下降的隶属度函数
        if x(k)>=xm(i,k)&&x(k)<=xm(i+1,k)
           ux(i,k)=0.5*sin(pi*(x(k)-xm(i,k))/abs(xm(i,k)-xm(i+1,k))+0.5*pi)+0.5; %一种具有一阶可导性的四边形家族隶属度函数
        end
    end
    for i=2:r  %从左到右只计算上升的隶属度函数
        if x(k)>=xm(i-1,k)&&x(k)<=xm(i,k)
           ux(i,k)=0.5*sin(pi*(x(k)-xm(i,k))/abs(xm(i-1,k)-xm(i,k))+0.5*pi)+0.5;
        end
    end
end

kx=1;
jz=1;
[beta,wdot]= fuzzyoutput(ux,x,xm,kx,jz);

% function  [Basic,beta]= sumfuzzy_test(x) 
% ux=x;
% im=1;
% jm=0;
% bias=1;
% Basic=0;
% dem=length(ux(:,1))^length(ux(1,:)); %隶属度函数的重数数量
% beta=zeros(dem,1);
% [Basic,beta] = myfun(im,jm,ux,bias,Basic,beta);
% function [Basic,beta,jm] = myfun(im,jm,ux,bias,Basic,beta) 
% %针对ux隶属度函数矩阵的中心平均解模糊，初值赋为1,0，ux，1，0，执行的是多重求和
%     if  im > length(ux(1,:))    %length(ux(1,:))为前件输入的维度
%         Basic = Basic + bias;
%         jm=jm+1;                %相对于i1...in规则编号，此处是从最后一列填满到第一列（i1,...,in）
%         beta(jm,1)=bias;        %beta(i1,...,in)*xk*z(i6,j)
%     else
%         for km=1:length(ux(:,1))   %length(ux(:,1))为规则数量
%             bias_last = bias;
%             bias = bias* ux(km,im);
%             im = im+1;
%             [Basic,beta,jm] = myfun(im,jm,ux,bias,Basic,beta); %递归，拦在这里一直到function执行结束,每执行一次就会多一个for循环（每次跳出就是再一次的for内循环）
%             im = im-1; 
%             bias  = bias_last;
%         end
%     end
% end


end

== matlab function DY05S600_robot_controller_main_opensource/ATS_controller/fuzzy_membership_function7 ==
  data: x input; beta output; wdot output
function [beta,wdot] = fcn(x)

%xm是规则中心
xm=zeros(5,4);
for j=1:5
    xm(j,1)=-0.26+0.13*(j-1)+0.1;
end
for j=6:10
    xm(j-5,2)=-0.18+0.09*(j-5-1)+0.1;
end
for j=11:15
    xm(j-10,3)=-0.14+0.07*(j-10-1)+0.1;
end
for j=16:20
    xm(j-15,4)=-0.4+0.2*(j-15-1)+0.1;
end


%xm是规则中心从小值到大值排列,x是前件变量,
r=length(xm(:,1)); %length(xm)是规则数量r
n=length(xm(1,:));%length(x)是前件变量维度
%初始化隶属度函数
ux=zeros(r,n);

for k=1:n
    if x(k)<=xm(1,k)   %论域左边界外
        ux(1,k)=1;
    end
    if x(k)>=xm(r,k)   %论域右边界外
        ux(r,k)=1;
    end
    for i=1:r-1  %从左到右只计算下降的隶属度函数
        if x(k)>=xm(i,k)&&x(k)<=xm(i+1,k)
           ux(i,k)=0.5*sin(pi*(x(k)-xm(i,k))/abs(xm(i,k)-xm(i+1,k))+0.5*pi)+0.5; %一种具有一阶可导性的四边形家族隶属度函数
        end
    end
    for i=2:r  %从左到右只计算上升的隶属度函数
        if x(k)>=xm(i-1,k)&&x(k)<=xm(i,k)
           ux(i,k)=0.5*sin(pi*(x(k)-xm(i,k))/abs(xm(i-1,k)-xm(i,k))+0.5*pi)+0.5;
        end
    end
end

kx=1;
jz=1;
[beta,wdot]= fuzzyoutput(ux,x,xm,kx,jz);

% function  [Basic,beta]= sumfuzzy_test(x) 
% ux=x;
% im=1;
% jm=0;
% bias=1;
% Basic=0;
% dem=length(ux(:,1))^length(ux(1,:)); %隶属度函数的重数数量
% beta=zeros(dem,1);
% [Basic,beta] = myfun(im,jm,ux,bias,Basic,beta);
% function [Basic,beta,jm] = myfun(im,jm,ux,bias,Basic,beta) 
% %针对ux隶属度函数矩阵的中心平均解模糊，初值赋为1,0，ux，1，0，执行的是多重求和
%     if  im > length(ux(1,:))    %length(ux(1,:))为前件输入的维度
%         Basic = Basic + bias;
%         jm=jm+1;                %相对于i1...in规则编号，此处是从最后一列填满到第一列（i1,...,in）
%         beta(jm,1)=bias;        %beta(i1,...,in)*xk*z(i6,j)
%     else
%         for km=1:length(ux(:,1))   %length(ux(:,1))为规则数量
%             bias_last = bias;
%             bias = bias* ux(km,im);
%             im = im+1;
%             [Basic,beta,jm] = myfun(im,jm,ux,bias,Basic,beta); %递归，拦在这里一直到function执行结束,每执行一次就会多一个for循环（每次跳出就是再一次的for内循环）
%             im = im-1; 
%             bias  = bias_last;
%         end
%     end
% end


end

== matlab function DY05S600_robot_controller_main_opensource/ATS_controller/fuzzy_membership_function8 ==
  data: x input; beta output; wdot output
function [beta,wdot] = fcn(x)

%xm是规则中心
xm=zeros(5,4);
for j=1:5
    xm(j,1)=-0.26+0.13*(j-1)+0.1;
end
for j=6:10
    xm(j-5,2)=-0.18+0.09*(j-5-1)+0.1;
end
for j=11:15
    xm(j-10,3)=-0.14+0.07*(j-10-1)+0.1;
end
for j=16:20
    xm(j-15,4)=-0.4+0.2*(j-15-1)+0.1;
end



%xm是规则中心从小值到大值排列,x是前件变量,
r=length(xm(:,1)); %length(xm)是规则数量r
n=length(xm(1,:));%length(x)是前件变量维度
%初始化隶属度函数
ux=zeros(r,n);

for k=1:n
    if x(k)<=xm(1,k)   %论域左边界外
        ux(1,k)=1;
    end
    if x(k)>=xm(r,k)   %论域右边界外
        ux(r,k)=1;
    end
    for i=1:r-1  %从左到右只计算下降的隶属度函数
        if x(k)>=xm(i,k)&&x(k)<=xm(i+1,k)
           ux(i,k)=0.5*sin(pi*(x(k)-xm(i,k))/abs(xm(i,k)-xm(i+1,k))+0.5*pi)+0.5; %一种具有一阶可导性的四边形家族隶属度函数
        end
    end
    for i=2:r  %从左到右只计算上升的隶属度函数
        if x(k)>=xm(i-1,k)&&x(k)<=xm(i,k)
           ux(i,k)=0.5*sin(pi*(x(k)-xm(i,k))/abs(xm(i-1,k)-xm(i,k))+0.5*pi)+0.5;
        end
    end
end

kx=1;
jz=1;
[beta,wdot]= fuzzyoutput(ux,x,xm,kx,jz);

% function  [Basic,beta]= sumfuzzy_test(x) 
% ux=x;
% im=1;
% jm=0;
% bias=1;
% Basic=0;
% dem=length(ux(:,1))^length(ux(1,:)); %隶属度函数的重数数量
% beta=zeros(dem,1);
% [Basic,beta] = myfun(im,jm,ux,bias,Basic,beta);
% function [Basic,beta,jm] = myfun(im,jm,ux,bias,Basic,beta) 
% %针对ux隶属度函数矩阵的中心平均解模糊，初值赋为1,0，ux，1，0，执行的是多重求和
%     if  im > length(ux(1,:))    %length(ux(1,:))为前件输入的维度
%         Basic = Basic + bias;
%         jm=jm+1;                %相对于i1...in规则编号，此处是从最后一列填满到第一列（i1,...,in）
%         beta(jm,1)=bias;        %beta(i1,...,in)*xk*z(i6,j)
%     else
%         for km=1:length(ux(:,1))   %length(ux(:,1))为规则数量
%             bias_last = bias;
%             bias = bias* ux(km,im);
%             im = im+1;
%             [Basic,beta,jm] = myfun(im,jm,ux,bias,Basic,beta); %递归，拦在这里一直到function执行结束,每执行一次就会多一个for循环（每次跳出就是再一次的for内循环）
%             im = im-1; 
%             bias  = bias_last;
%         end
%     end
% end


end

== matlab function DY05S600_robot_controller_main_opensource/ATS_controller/TSfuzzy_system_output10 ==
  data: beta input; w input; AF11 output
function AF11  = fcn(beta,w)

AF11=0;
for i=1:length(beta)
    AF11=AF11+w(i,1)*beta(i,1);
end

end

== matlab function DY05S600_robot_controller_main_opensource/ATS_controller/TSfuzzy_system_output11 ==
  data: beta input; w input; AF11 output
function AF11  = fcn(beta,w)

AF11=0;
for i=1:length(beta)
    AF11=AF11+w(i,1)*beta(i,1);
end

end

== matlab function DY05S600_robot_controller_main_opensource/ATS_controller/TSfuzzy_system_output12 ==
  data: beta input; w input; AF11 output
function AF11  = fcn(beta,w)

AF11=0;
for i=1:length(beta)
    AF11=AF11+w(i,1)*beta(i,1);
end

end

== matlab function DY05S600_robot_controller_main_opensource/ATS_controller/TSfuzzy_system_output9 ==
  data: beta input; w input; AF11 output
function AF11  = fcn(beta,w)

AF11=0;
for i=1:length(beta)
    AF11=AF11+w(i,1)*beta(i,1);
end

end

== matlab function DY05S600_robot_controller_main_opensource/ATS_controller/controller3 ==
  data: AF11 input; AF12 input; AF21 input; AF22 input; K1 input; K2 input; u1 output; u2 output; x1 input; x2 input; dag output
function [u1,u2,dag]  = fcn(AF11,AF12,AF21,AF22,K1,K2,x1,x2)

b1=0.1;
b2=0.01;

dag=1.3*pi/180;

% u1=-1/b1*((0+AF11)*x1+(0+AF12)*x2+K1*x1/dag^2);
% 
% u2=-1/b2*((0+AF21)*x1+(0+AF22)*x2+K2*x2/dag^2);

% dagx1=0.5*pi/180;
% satx1=0;
% if abs(x1)<dagx1
%     satx1=sign(x1);
% else
%     satx1=x1/dagx1;
% end

   
u1=-1/b1*((0.6+AF11)*x1+(0+AF12)*x2+K1*4/pi*atan(x1/dag));

u2=-1/b2*((2+AF21)*x1+(0.6+AF22)*x2+K2*4/pi*atan(x2/dag));


end

== matlab function DY05S600_robot_controller_main_opensource/ATS_controller/fuzzy_membership_function10 ==
  data: x input; beta output; wdot output
function [beta,wdot] = fcn(x)

%xm是规则中心
xm=zeros(5,4);
for j=1:5
    xm(j,1)=-0.26+0.13*(j-1)+0.1;
end
for j=6:10
    xm(j-5,2)=-0.18+0.09*(j-5-1)+0.1;
end
for j=11:15
    xm(j-10,3)=-0.14+0.07*(j-10-1)+0.1;
end
for j=16:20
    xm(j-15,4)=-0.4+0.2*(j-15-1)+0.1;
end



%xm是规则中心从小值到大值排列,x是前件变量,
r=length(xm(:,1)); %length(xm)是规则数量r
n=length(xm(1,:));%length(x)是前件变量维度
%初始化隶属度函数
ux=zeros(r,n);

for k=1:n
    if x(k)<=xm(1,k)   %论域左边界外
        ux(1,k)=1;
    end
    if x(k)>=xm(r,k)   %论域右边界外
        ux(r,k)=1;
    end
    for i=1:r-1  %从左到右只计算下降的隶属度函数
        if x(k)>=xm(i,k)&&x(k)<=xm(i+1,k)
           ux(i,k)=0.5*sin(pi*(x(k)-xm(i,k))/abs(xm(i,k)-xm(i+1,k))+0.5*pi)+0.5; %一种具有一阶可导性的四边形家族隶属度函数
        end
    end
    for i=2:r  %从左到右只计算上升的隶属度函数
        if x(k)>=xm(i-1,k)&&x(k)<=xm(i,k)
           ux(i,k)=0.5*sin(pi*(x(k)-xm(i,k))/abs(xm(i-1,k)-xm(i,k))+0.5*pi)+0.5;
        end
    end
end

kx=1;
jz=1;
[beta,wdot]= fuzzyoutput(ux,x,xm,kx,jz);

% function  [Basic,beta]= sumfuzzy_test(x) 
% ux=x;
% im=1;
% jm=0;
% bias=1;
% Basic=0;
% dem=length(ux(:,1))^length(ux(1,:)); %隶属度函数的重数数量
% beta=zeros(dem,1);
% [Basic,beta] = myfun(im,jm,ux,bias,Basic,beta);
% function [Basic,beta,jm] = myfun(im,jm,ux,bias,Basic,beta) 
% %针对ux隶属度函数矩阵的中心平均解模糊，初值赋为1,0，ux，1，0，执行的是多重求和
%     if  im > length(ux(1,:))    %length(ux(1,:))为前件输入的维度
%         Basic = Basic + bias;
%         jm=jm+1;                %相对于i1...in规则编号，此处是从最后一列填满到第一列（i1,...,in）
%         beta(jm,1)=bias;        %beta(i1,...,in)*xk*z(i6,j)
%     else
%         for km=1:length(ux(:,1))   %length(ux(:,1))为规则数量
%             bias_last = bias;
%             bias = bias* ux(km,im);
%             im = im+1;
%             [Basic,beta,jm] = myfun(im,jm,ux,bias,Basic,beta); %递归，拦在这里一直到function执行结束,每执行一次就会多一个for循环（每次跳出就是再一次的for内循环）
%             im = im-1; 
%             bias  = bias_last;
%         end
%     end
% end


end

== matlab function DY05S600_robot_controller_main_opensource/ATS_controller/fuzzy_membership_function11 ==
  data: x input; beta output; wdot output
function [beta,wdot] = fcn(x)

%xm是规则中心
xm=zeros(5,4);
for j=1:5
    xm(j,1)=-0.26+0.13*(j-1)+0.1;
end
for j=6:10
    xm(j-5,2)=-0.18+0.09*(j-5-1)+0.1;
end
for j=11:15
    xm(j-10,3)=-0.14+0.07*(j-10-1)+0.1;
end
for j=16:20
    xm(j-15,4)=-0.4+0.2*(j-15-1)+0.1;
end


%xm是规则中心从小值到大值排列,x是前件变量,
r=length(xm(:,1)); %length(xm)是规则数量r
n=length(xm(1,:));%length(x)是前件变量维度
%初始化隶属度函数
ux=zeros(r,n);

for k=1:n
    if x(k)<=xm(1,k)   %论域左边界外
        ux(1,k)=1;
    end
    if x(k)>=xm(r,k)   %论域右边界外
        ux(r,k)=1;
    end
    for i=1:r-1  %从左到右只计算下降的隶属度函数
        if x(k)>=xm(i,k)&&x(k)<=xm(i+1,k)
           ux(i,k)=0.5*sin(pi*(x(k)-xm(i,k))/abs(xm(i,k)-xm(i+1,k))+0.5*pi)+0.5; %一种具有一阶可导性的四边形家族隶属度函数
        end
    end
    for i=2:r  %从左到右只计算上升的隶属度函数
        if x(k)>=xm(i-1,k)&&x(k)<=xm(i,k)
           ux(i,k)=0.5*sin(pi*(x(k)-xm(i,k))/abs(xm(i-1,k)-xm(i,k))+0.5*pi)+0.5;
        end
    end
end

kx=1;
jz=1;
[beta,wdot]= fuzzyoutput(ux,x,xm,kx,jz);

% function  [Basic,beta]= sumfuzzy_test(x) 
% ux=x;
% im=1;
% jm=0;
% bias=1;
% Basic=0;
% dem=length(ux(:,1))^length(ux(1,:)); %隶属度函数的重数数量
% beta=zeros(dem,1);
% [Basic,beta] = myfun(im,jm,ux,bias,Basic,beta);
% function [Basic,beta,jm] = myfun(im,jm,ux,bias,Basic,beta) 
% %针对ux隶属度函数矩阵的中心平均解模糊，初值赋为1,0，ux，1，0，执行的是多重求和
%     if  im > length(ux(1,:))    %length(ux(1,:))为前件输入的维度
%         Basic = Basic + bias;
%         jm=jm+1;                %相对于i1...in规则编号，此处是从最后一列填满到第一列（i1,...,in）
%         beta(jm,1)=bias;        %beta(i1,...,in)*xk*z(i6,j)
%     else
%         for km=1:length(ux(:,1))   %length(ux(:,1))为规则数量
%             bias_last = bias;
%             bias = bias* ux(km,im);
%             im = im+1;
%             [Basic,beta,jm] = myfun(im,jm,ux,bias,Basic,beta); %递归，拦在这里一直到function执行结束,每执行一次就会多一个for循环（每次跳出就是再一次的for内循环）
%             im = im-1; 
%             bias  = bias_last;
%         end
%     end
% end


end
